simulink model "Practice_04_model"  (R2024b)
settings: Solver=VariableStepAuto  StartTime=0.0  StopTime=stopTime  RelTol=1e-3
values from neighbouring files (symbols this model uses):
  alpha_mu = 50/10*9    (= 45)    [Practice_04_script.m]
  beta_mu = 50    [Practice_04_script.m]
  m = mean(x)    [computeMCstats.m]
undefined symbols (not defined in the file or in its folder): n
settings Model: SimulationMode=accelerator  Creator=Dario  LastModifiedBy=Lorenzo
settings DataIOCC: SaveOperatingPoint=on
settings DebuggingCC: UnconnectedInputMsg=warning  UnconnectedOutputMsg=warning  UnconnectedLineMsg=warning
settings ModelReferenceCC: EnableRefExpFcnMdlSchedulingChecks=on
settings RTWCC: GPUComputeCapability=3.5  DLArmComputeVersion=19.05

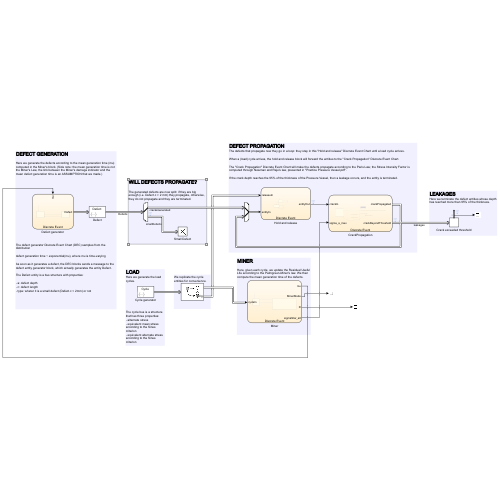
[thumbnail: Simulink's stored preview of the top-level diagram]
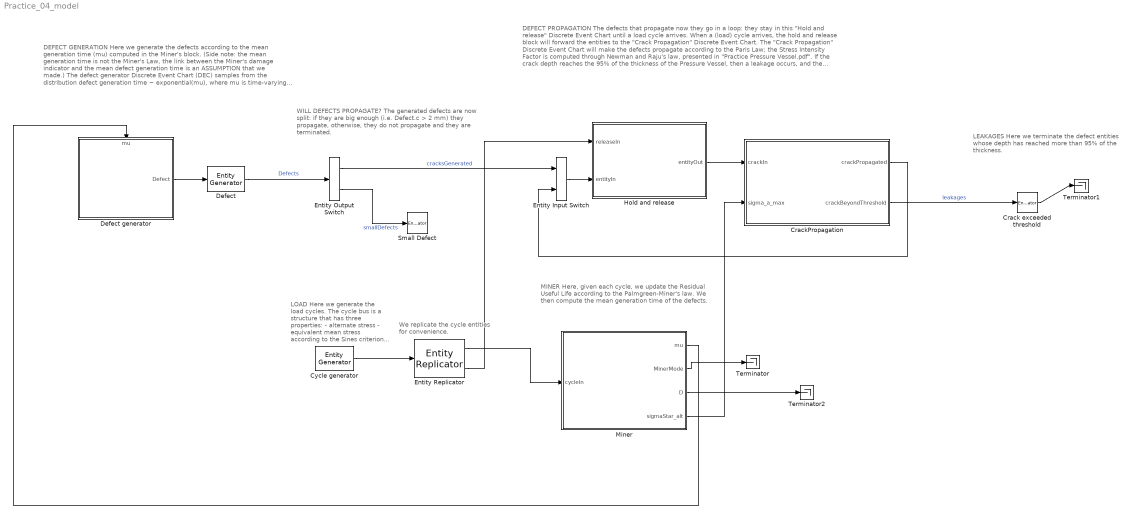
== system Practice_04_model ==
  note: LOAD
      | Here we generate the load cycles.
      |
      | The cycle bus is a structure that has three properties:
      | - alternate stress
      | - equivalent mean stress according to the Sines criterion
      | - equivalent alternate stress according to the Sines criterion
  note: We replicate the cycle entities for convenience.
  note: MINER
      |
      | Here, given each cycle, we update the Residual Useful Life according to the Palmgreen-Miner's law. We then compute the mean generation time of the defects.
  note: DEFECT GENERATION
      |
      | Here we generate the defects according to the mean generation time (mu) computed in the Miner's block. (Side note: the mean generation time is not the Miner's Law, the link between the Miner's damage indicator and the mean defect generation time is an ASSUMPTION that we made.)
      |
      | The defect generator Discrete Event Chart (DEC) samples from the distribution
      |
      | defect generation time ~ exponential(mu), where mu is time-varying
      |
      | As soon as it generates a defect, the DEC blocks sends a message to the defect entity generator block, which actually generates the entity Defect.
      |
      | The Defect entity is a bus structure with properties:
      |
      | - a: defect depth
      | - c: defect length
      | - type: wheter it is a small defect (Defect.c < 2mm) or not
  note: WILL DEFECTS PROPAGATE?
      |
      | The generated defects are now split: if they are big enough (i.e. Defect.c > 2 mm) they propagate, otherwise, they do not propagate and they are terminated.
  note: DEFECT PROPAGATION
      | The defects that propagate now they go in a loop: they stay in this "Hold and release" Discrete Event Chart until a load cycle arrives.
      |
      | When a (load) cycle arrives, the hold and release block will forward the entities to the "Crack Propagation" Discrete Event Chart.
      |
      | The "Crack Propagation" Discrete Event Chart will make the defects propagate according to the Paris Law; the Stress Intensity Factor is computed through Newman and Raju's law, presented in "Practice Pressure Vessel.pdf".
      |
      | If the crack depth reaches the 95% of the thickness of the Pressure Vessel, then a leakage occurs, and the entity is terminated.
  note: LEAKAGES
      | Here we terminate the defect entities whose depth has reached more than 95% of the thickness.
  Crack exceeded threshold : EntityTerminator  InputPortMessageModes=m  NumberEntitiesArrived=on
      settings: OutputPortMap=o0
  CrackPropagation : Stateflow chart  TreatAsAtomicUnit=on
  Cycle generator : EntityGenerator  OutputPortMessageModes=m  Period=24  GenerateAction=|  AttributeName=deltaSigma|sigmaStar_alt|sigmaStar_mean  AttributeInitialValue=1|1|1  EntityType=Bus object  EntityTypeName=Cycle
      | % entity.deltaSigma = 20 + randn; % [MPa]
      | % C = cycleStorage.data.sigmaStar_alt/(1-cycleStorage.data.sigmaStar_mean/UTS);
      | persistent init
      | if isempty(init)
      |     rng(seed+236845);
      | end
      | p = 21 + randn; % [MPa] % It should be 20 by design
      | Dm = 230;
      | t = 3.2;
      | sigma_a_alt = p*Dm/(4*t)/2;
      | sigma_a_mean = sigma_a_alt;
      | sigma_theta_alt = p*Dm/(2*t)/2;
      | sigma_theta_mean = sigma_theta_alt; 
      | entity.sigma_a_max = sigma_a_alt*2; 
      | entity.sigmaStar_alt = sqrt(sigma_a_alt^2 + sigma_theta_alt^2 - sigma_a_alt*sigma_theta_alt);
      | entity.sigmaStar_mean = sigma_a_mean + sigma_theta_mean;
  Defect : EntityGenerator  InputPortMessageModes=m  OutputPortMessageModes=m  GenerationMethod=Event-based  GenerateAction=|  AttributeName=size|type  AttributeInitialValue=0|1  EntityType=Bus object  EntityTypeName=Defect
      | persistent init
      | if isempty(init)
      |     init = 1;
      |     entity.c = wblrnd(3, 2);% [mm]
      |     entity.a = entity.c/5;
      |     rng(seed+12354);
      | else
      |     entity.c = wblrnd(3, 2);% [mm]
      |     entity.a = entity.c/5;
      | end
      | if entity.c > 2;
      |     entity.type = 1; % Crack
      | else
      |     entity.type = 2; % Defect
      | end
      settings: InputPortMap=u0
  Defect generator : Stateflow chart  TreatAsAtomicUnit=on
      settings: PortSchema="{\"entries\":[{\"content\":{\"sides\":[{\"content\":{\"connectorIds\":[]},\"type\":\"ConnectorPlacement.EquallySpacedRectSide\",\"uuid\":\"142f5b06-4bf9-426f-8771-5ff0a5bbac91\"},{\"content\":{\"connectorIds\":[\"Out1\"],\"side\":\"RIGHT\"},\"type\":\"ConnectorPlacement.EquallySpacedRectSide\",\"uuid\":\"5b0d92c9-c6d8-4539-adfd-0bac753e5bde\"},{\"content\":{\"connectorIds\":[\"In1\"],\"side\":\"TOP\"},\"type\":\"ConnectorPlacement.EquallySpacedRectSide\",\"uuid\":\"f71819d8-dd85-4027-9822-23ffe5b01f2f\"}]},\"type\":\"ConnectorPlacement.EquallySpacedConnector\",\"uuid\":\"09995b11-d41e-4af5-9da5-428be56c701e\"}],\"packageUris\":[\"http://schema.mathworks.com/mf0/Connector/R2020b\"],\"version\":\"1.0\"}"
  Entity Input Switch : EntityInputSwitch  InputPortMessageModes=m,m  OutputPortMessageModes=m
  Entity Output Switch : EntityOutputSwitch  InputPortMessageModes=m  OutputPortMessageModes=m,m  SwitchingCriterion=From attribute  SwitchAttributeName=type
  Entity Replicator : EntityReplicator  InputPortMessageModes=m  OutputPortMessageModes=m,m
  Hold and release : Stateflow chart  TreatAsAtomicUnit=on
  Miner : Stateflow chart  TreatAsAtomicUnit=on
  Small Defect : EntityTerminator  InputPortMessageModes=m
  Terminator : Terminator
  Terminator1 : Terminator
  Terminator2 : Terminator
  wires:
  Miner/1(mu) -> Defect generator/1(mu)
  Defect generator/1(Defect) -> Defect/1
  Cycle generator/1 -> Entity Replicator/1
  Defect/1 -> Entity Output Switch/1  "Defects"
  Miner/2(MinerMode) -> Terminator/1
  Entity Output Switch/2 -> Small Defect/1  "smallDefects"
  Entity Input Switch/1 -> Hold and release/2(entityIn)
  Entity Replicator/1 -> Miner/1(cycleIn)
  Entity Replicator/2 -> Hold and release/1(releaseIn)
  Entity Output Switch/1 -> Entity Input Switch/1  "cracksGenerated"
  Hold and release/1(entityOut) -> CrackPropagation/1(crackIn)
  CrackPropagation/2(crackBeyondThreshold) -> Crack exceeded threshold/1  "leakages"
  CrackPropagation/1(crackPropagated) -> Entity Input Switch/2
  Miner/4(sigmaStar_alt) -> CrackPropagation/2(sigma_a_max)
  Crack exceeded threshold/1 -> Terminator1/1
  Miner/3(D) -> Terminator2/1

== stateflow chart Practice_04_model/CrackPropagation ==
  settings: enableNonTerminalStates=1
  note: Whenever an entity arrives
  state Idle
  note: We receive it, and compute the stress intensity factor according to the SIF function, which implements the Newman and Raju's law. Then we propagate the crack in both directions using the Paris Law
  note: If the crack depth is above 95% of the Vessel Thickness
  note: If the crack depth is below the 95% of the thickness
  note: Forward the entity to the crackBeyondThreshold output port
  note: Forward the entity to the CrackPropagated output port
  (default) -> Idle
  Idle -> (junction 25) : crackIn{forward(crackIn, crackStorage)}
  (junction 25) -> (junction 27) : {receive(crackStorage)
      | K_a = SIF(3.2, 100, crackStorage.data.a, crackStorage.data.c, pi/2, sigma_a_max, 0);
      | crackStorage.data.a = crackStorage.data.a + C*K_a^(m);
      | K_c = SIF(3.2, 100, crackStorage.data.a, crackStorage.data.c, 0, sigma_a_max, 0);
      | crackStorage.data.c = crackStorage.data.c + C*K_c^(m);
      | %disp('crackStorage.data.a')
      | %disp(crackStorage.data.a)
      | }
  (junction 27) -> (junction 45) [order 1] : [crackStorage.data.a >= 0.95*3.2]
  (junction 45) -> (junction 47) : {forward(crackStorage, crackBeyondThreshold);}
  (junction 27) -> (junction 51) [order 2] : [crackStorage.data.a < 0.95*3.2]
  (junction 47) -> Idle
  (junction 51) -> (junction 47) : {forward(crackStorage, crackPropagated);}
  data: t function_input; w function_input; a function_input; c function_input; phi function_input; St function_input; Sb function_input; K function_output; crackPropagated output Bus: Defect; crackIn input Bus: Defect; crackBeyondThreshold output Bus: Defect; C constant double =2.5e-13; m constant double =3; K_a local; K_c local; crackStorage local Bus: Defect; sigma_a_max input
  function K = SIF(t,w,a,c,phi,St,Sb):
    | function K = SIF(t,w,a,c,phi,St,Sb)
    | 
    | ac=a/c;
    | at=a/t;   
    | 
    | M1=1.13-0.09*ac;
    | M2=-0.54+0.89/(0.2+ac);
    | M3=0.5-1/(0.65+ac)+14*(1-ac)^24;
    | 
    | g=1+(0.1+0.35*at^2)*(1-sin(phi))^2;
    | fp=(ac^2*(cos(phi))^2+(sin(phi))^2)^0.25;
    | fw=sqrt(sec(pi*c/2/w*sqrt(at)));
    | 
    | F=(M1+M2*at^2+M3*at^4)*g*fp*fw;
    | 
    | Q=1+1.464*ac^1.65;
    | 
    | p=0.2+ac+0.6*at;
    | H1=1-0.34*at-0.11*ac*at;
    | G1=-1.22-0.12*ac;
    | G2=0.55-1.05*ac^0.75+0.47*ac^1.5;
    | H2=1+G1*at+G2*at^2;
    | H=H1+(H2-H1)*(sin(phi))^p;
    | 
    | K=(St+H*Sb)*sqrt(pi*a/Q)*F;
    | 
    | return

== stateflow chart Practice_04_model/Miner ==
  settings: enableNonTerminalStates=1
  note: Whenever a cycle arrives, we go into the Cycle state
  state Idle
  state Cycle
    entry:
    receive(cycleStorage)
    Cstar = cycleStorage.data.sigmaStar_alt/(1-cycleStorage.data.sigmaStar_mean/UTS); % Constant defined for convenience
    sigmaStar_alt =  cycleStorage.data.sigmaStar_alt; % We extract the property from the cycle entity
    N = 10^(log10(Cstar/A)*1/b); % Number of cycles to failure due to the cycle entity that has arrived.
    D = D + 1/N; % Miner Damage indicator
    mu = beta_mu - D * alpha_mu; % We compute the inter generation time
    if mu < 1
    mu = 1;
    end
    if D >= 1;
    D = 1; % No more RUL according to Miner
    %disp('noMoreRUL')
    end
    end
  (default) -> Idle : {D = 0;
      | mu = 100;}
  Idle -> Cycle : cycleIn{forward(cycleIn, cycleStorage)}
  Cycle -> Idle
  data: cycleStorage local Bus: Cycle; cycleIn input Bus: Cycle; b constant double size=1 =-0.107581301877432; N local; A constant double =1892.28442620405; UTS constant double =1000; Cstar local; mu output; MinerMode output Enum: MinerModeType; D output =0; sigmaStar_alt output; alpha_mu parameter; beta_mu parameter

== stateflow chart Practice_04_model/Defect generator ==
  settings: enableNonTerminalStates=1
  note: We generate an output message and send it after the time sampled from the exponential distribution with mu as mean time to generation
  state Idle
  state Generation
  (default) -> Idle : {rng(seed+35468)} % We set the seed at the start of the simulation
  Idle -> Generation : after(exprnd(mu), sec){Defect.data = 1; send(Defect);}
  Generation -> Idle
  data: Defect output; mu input; seed parameter double

== stateflow chart Practice_04_model/Hold and release ==
  settings: enableNonTerminalStates=1
  note: Whenever a crack arrives, we put it in the storage
  state Idle
  note: When entityStorage is empty, we transition to Idle after 0.01 time units
  note: Whenever a cycle (releaseIn) arrives, we go into the Forwarding state
  state Forwarding
    %entry:
    %discard(releaseIn)
    %disp(length(entityStorage))%
    %end
  note: If entityStorage contains at least one entity, we forward it to entityOut (It is basically a loop)
  note: releaseIn{disp('Length entity storage');disp(length(entityStorage));}
  (default) -> Idle
  Idle -> (junction 7) [order 1] : entityIn
  (junction 7) -> (junction 9) : {forward(entityIn, entityStorage);}
  Forwarding -> Idle [order 2] : after(0.01, sec)
  (junction 9) -> Idle
  Idle -> Forwarding [order 2] : releaseIn
  Forwarding -> (junction 16) [order 1] : entityStorage
  (junction 16) -> (junction 18) : {forward(entityStorage, entityOut);}
  (junction 18) -> Forwarding
  data: entityStorage local Bus: Defect; releaseIn input Bus: Cycle; entityIn input Bus: Defect; entityOut output Bus: Defect
